simulink model "sim_Pendulum_withFreeSupport"  (R2020a)
settings: Solver=VariableStepAuto  StartTime=0.0  StopTime=t_sim  MaxStep=0.1  RelTol=1e-3
values from neighbouring files (symbols this model uses):
  g = 9.81    [Pendulum_TrolleyWithSwingingLoad.m]    (also in Pendulum_withFreeSupport.m = 9.8)
  l = 4    [Pendulum_TrolleyWithSwingingLoad.m]    (also in Pendulum_withFreeSupport.m = 10)
  m = 200    [Pendulum_withFreeSupport.m]
  M = feedback(Gc*Gp, H)    [PIDController_eg2.m]    (also in Pendulum_withFreeSupport.m = 400)
  theta0_rad = (pi/180)*theta0    (= 0.523598775598)    [Pendulum_withFreeSupport.m]
  v0 = 6    [Pendulum_withFreeSupport.m]
settings Model: Creator=Samir  LastModifiedBy=Samir

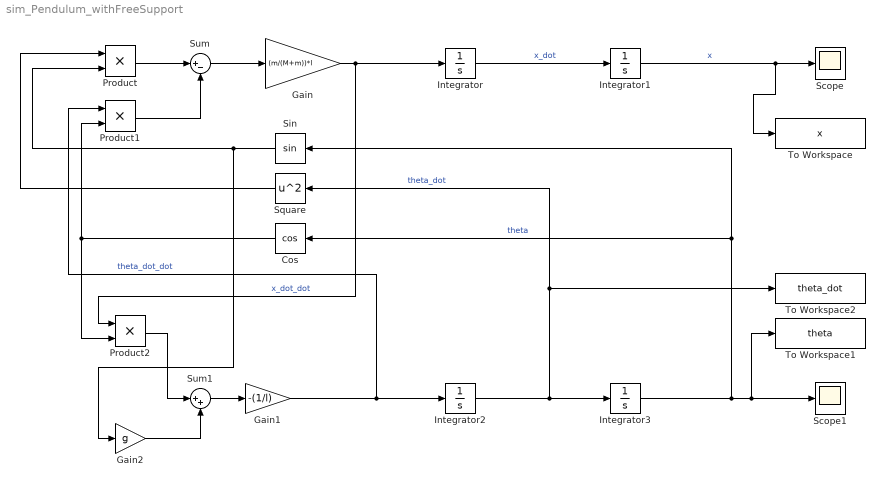
== system sim_Pendulum_withFreeSupport ==
  Cos : Trigonometry  Operator=cos
  Gain : Gain  Gain=(m/(M+m))*l
  Gain1 : Gain  Gain=-(1/l)
  Gain2 : Gain  Gain=g
  Integrator : Integrator  InitialCondition=v0
  Integrator1 : Integrator
  Integrator2 : Integrator
  Integrator3 : Integrator  InitialCondition=theta0_rad
  Product : Product
  Product1 : Product
  Product2 : Product
  Scope : Scope
  Scope1 : Scope
  Sin : Trigonometry
  Square : Math  Operator=square  SaturateOnIntegerOverflow=on
  Sum : Sum  Inputs=|+-
  Sum1 : Sum  Inputs=|++
  To Workspace : ToWorkspace  VariableName=x  SaveFormat=Timeseries  SampleTime=-1
  To Workspace1 : ToWorkspace  VariableName=theta  SaveFormat=Timeseries  SampleTime=-1
  To Workspace2 : ToWorkspace  VariableName=theta_dot  SaveFormat=Timeseries  SampleTime=-1
  wires:
  Integrator/1 -> Integrator1/1  "x_dot"
  Integrator1/1 -> To Workspace/1, Scope/1  "x"
  Gain/1 -> Product2/1, Integrator/1  "x_dot_dot"
  Gain1/1 -> Product1/1, Integrator2/1  "theta_dot_dot"
  Integrator3/1 -> Cos/1, Sin/1, Scope1/1, To Workspace1/1  "theta"
  Integrator2/1 -> To Workspace2/1, Square/1, Integrator3/1  "theta_dot"
  Sum/1 -> Gain/1
  Product/1 -> Sum/1
  Square/1 -> Product/1
  Sin/1 -> Gain2/1, Product/2
  Product1/1 -> Sum/2
  Cos/1 -> Product2/2, Product1/2
  Sum1/1 -> Gain1/1
  Gain2/1 -> Sum1/2
  Product2/1 -> Sum1/1
